simulink model "Model"  (R2016a)
settings: Solver=ode3  SolverMode=SingleTasking  StartTime=0.0  StopTime=inf  FixedStep=0.005  RelTol=1e-3
StartFcn:
  | clear functions
settings Model: Creator=Edin Koco  LastModifiedBy=Zvonimir
settings DataIOCC: LimitDataPoints=on  SaveFormat=Array
settings DebuggingCC: UnderspecifiedInitializationDetection=Classic  MergeDetectMultiDrivingBlocksExec=none  SolverPrmCheckMsg=warning  StateNameClashWarn=warning
settings HardwareCC: ProdBitPerPointer=32  ProdLargestAtomicFloat=None  ProdIntDivRoundTo=Undefined  ProdEndianess=Unspecified  ProdWordSize=32  ProdHWDeviceType=32-bit Generic
settings ModelReferenceCC: PropagateSignalLabelsOutOfModel=off
settings ConfigComp: CovModelRefEnable=Off

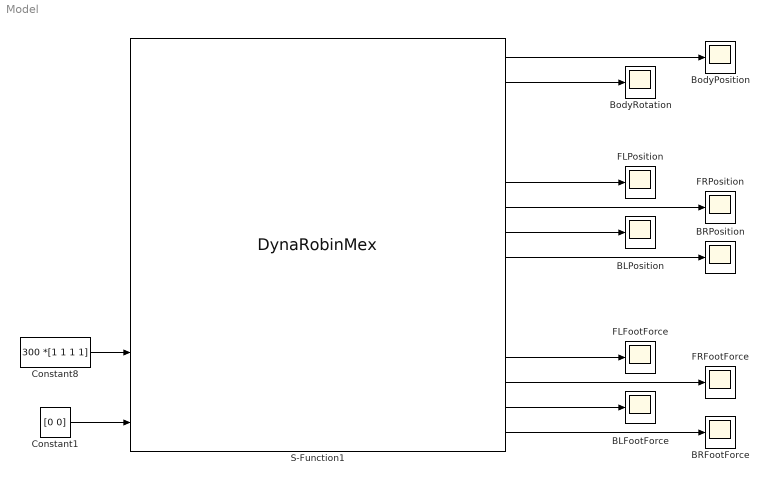
== system Model ==
  BLFootForce : Scope
  BLPosition : Scope
  BRFootForce : Scope
  BRPosition : Scope
  BodyPosition : Scope
  BodyRotation : Scope
  Constant1 : Constant  Value=[0 0]
  Constant8 : Constant  Value=300 *[1 1 1 1]
  FLFootForce : Scope
  FLPosition : Scope
  FRFootForce : Scope
  FRPosition : Scope
  S-Function1 : S-Function  FunctionName=DynaRobinMex  Parameters=0.005 0 0  SFunctionDeploymentMode=off  EnableBusSupport=off
  wires:
  Constant1/1 -> S-Function1/6
  S-Function1/2 -> BodyRotation/1
  S-Function1/1 -> BodyPosition/1
  S-Function1/9 -> BRPosition/1
  S-Function1/8 -> BLPosition/1
  S-Function1/7 -> FRPosition/1
  S-Function1/6 -> FLPosition/1
  Constant8/1 -> S-Function1/5
  S-Function1/16 -> BRFootForce/1
  S-Function1/15 -> BLFootForce/1
  S-Function1/14 -> FRFootForce/1
  S-Function1/13 -> FLFootForce/1
  ? -> S-Function1/1
  ? -> S-Function1/2
  ? -> S-Function1/3
  ? -> S-Function1/4
